simulink model "bola_viga_V_REP_Simulink"  (R2018a)
settings: Solver=ode45  StartTime=0.0  StopTime=144  RelTol=1e-3  EnableMultiTasking=on
undefined symbols (not defined in the file or in its folder): AD, BD, CD, K1, L1, Rep, T, V, V_Rep
libraries: simulink x2, aerolibanimutils x2
settings Model: Creator=HAROLD  LastModifiedBy=HAROLD
settings DataIOCC: LimitDataPoints=on  SaveFormat=Array
settings OptimizationCC: LifeSpan=inf
settings DebuggingCC: SFUnexpectedBacktrackingDiag=warning  SFNoUnconditionalDefaultTransitionDiag=warning  SFExecutionAtInitializationDiag=none
settings HardwareCC: ProdBitPerPointer=32  ProdBitPerSizeT=32  ProdBitPerPtrDiffT=32  ProdLargestAtomicFloat=None  ProdIntDivRoundTo=Undefined  ProdEndianess=Unspecified  ProdWordSize=32  ProdHWDeviceType=32-bit Generic
settings ModelReferenceCC: PropagateSignalLabelsOutOfModel=off
settings CodeAppCC: StateflowObjectComments=on
settings GRTTargetCC: TargetLangStandard=C89/C90 (ANSI)  GeneratePreprocessorConditionals=Disable all
settings ConfigComp: CovMetricSettings=dw  CovHtmlReporting=on  CovSaveCumulativeToWorkspaceVar=on  CovSaveSingleToWorkspaceVar=on  CovExternalEMLEnable=off

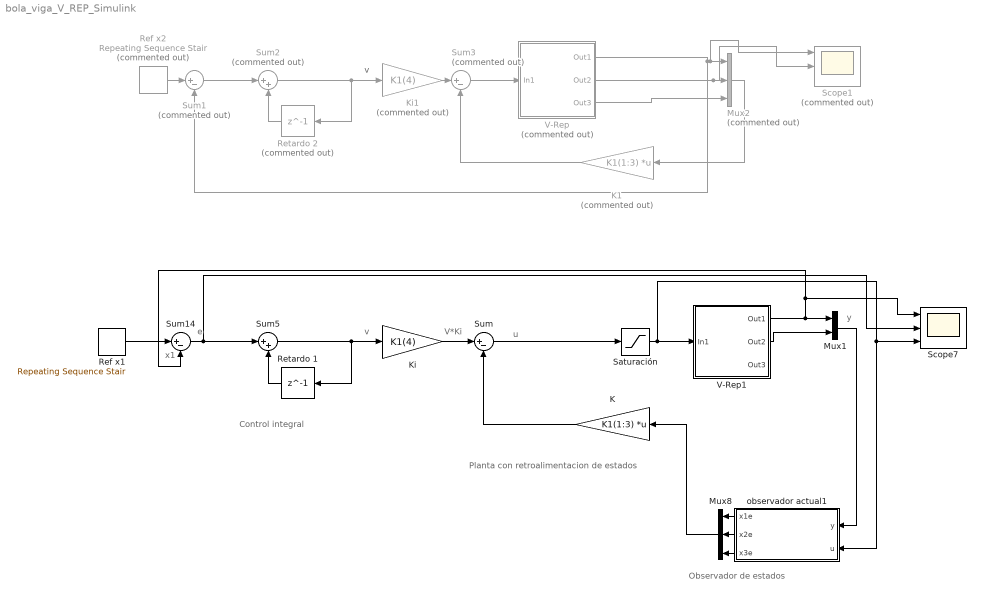
== system bola_viga_V_REP_Simulink ==
  note: v
  note: x1
  note: V*Ki
  note: y
  note: u
  note: v
  note: e
  note: Planta con retroalimentacion de estados
  note: Control integral
  note: Observador de estados
  K : Gain  Gain=K1(1:3)  Multiplication=Matrix(K*u)
  K1 : Gain  Commented=on  Gain=K1(1:3)  Multiplication=Matrix(K*u)
  Ki : Gain  Gain=K1(4)
  Ki1 : Gain  Commented=on  Gain=K1(4)
  Mux1 : Mux  Inputs=2
  Mux2 : Mux  Commented=on  Inputs=3
  Mux8 : Mux  Inputs=3
  Ref x1 : simulink/Sources/Repeating Sequence Stair  OutValues="[0  0.4 -0.4 -0.1 -0.3].'"  tsamp=36*0.8  OutMin=[]  OutMax=[]  OutDataTypeStr=double  OutputDataTypeScalingMode=double  OutDataType=fixdt(0,8)  ConRadixGroup=Best Precision: Vector-wise  OutScaling=2^-12
  Ref x2 : simulink/Sources/Repeating Sequence Stair  Commented=on  OutValues="[0.2  0.4 -0.4 -0.1 -0.3].'"  tsamp=36  OutMin=[]  OutMax=[]  OutDataTypeStr=double  OutputDataTypeScalingMode=double  OutDataType=fixdt(0,8)  ConRadixGroup=Best Precision: Vector-wise  OutScaling=2^-12
  Retardo 1 : Delay  DelayLength=1  SampleTime=T
  Retardo 2 : Delay  Commented=on  DelayLength=1  SampleTime=T
  Saturación : Saturate  UpperLimit=2.11  LowerLimit=-2.11
  Scope1 : Scope  Commented=on  NumInputPorts=3
  Scope7 : Scope  NumInputPorts=3
  Sum : Sum  Inputs=|+-
  Sum1 : Sum  Commented=on  Inputs=|+-
  Sum14 : Sum  Inputs=|+-
  Sum2 : Sum  Commented=on  Inputs=|++
  Sum3 : Sum  Commented=on  Inputs=|+-
  Sum5 : Sum  Inputs=|++
  V-Rep : Subsystem  Commented=on  AncestorBlock=V_Rep/V-Rep  mask(Bloque de V_Rep){Directory=Por Defecto, Parameter1=Bola Viga, Parameter2=T, Parameter3=2, Parameter6=off, Parameter7=3, Parameter8=C:\Program Files\V-REP3\V-REP_PRO_EDU}
      mask prompts: Directory "Directorio de V-Rep"; Parameter1 "Planta a emular"; Parameter2 "Tiempo de muestreo"; Parameter3 "sfdhg"; Parameter6 "Mostrar error de paso"; Parameter7 "Numero de salidas"; Parameter8 "dasads"
      mask help: Este bloque realiza una conexión con V_Rep, teniendo unas plantas ya preprogramadas para su mayor facilidad.
      mask init:
      | switch get_param(gcb,'Parameter1');
      |     case 'Péndulo de Furuta'
      |         t='3';
      |     case 'Bola Plato'
      |         t='1';
      |     case 'Bola Viga'
      |         t='2';
      |     case 'Otros'
      |         t='0';
      | end
      | set_param(gcb,'Parameter3',t);
      mask TypeOptions Directory: Por Defecto | C:\Program Files\V-REP3\V-REP_PRO_EDU
      mask Callback Directory:
      | DIR=get_param(gcb,'Directory');
      | 
      | if(strcmpi(DIR,'Por Defecto'));
      |     if ismac
      |         DIR='/Applications/V-REP_PRO_EDU_V3_6_2_Mac';
      |     elseif ispc
      |         DIR='C:\Program Files\V-REP3\V-REP_PRO_EDU'
      |     end
      | 
      | end
      | 
      | if ~strcmp(DIR,get_param(gcb,'Parameter8'))
      |     if ~exist(DIR, 'dir')
      |         baseException = MException('MYFUN:BadIndex','MYFUN:BadIndex');
      |         throw(baseException);
      |     else
      | 
      |         if~exist(strcat(DIR,'/credits.txt'), 'file')
      |            baseException = MException('MYFUN:BadIndex','V-Rep no está instalado en el directorio indicado');
      |            throw(baseException);
      |         else
      | 
      |             assignin('base','Path', {['-I' DIR '/programming/common/'],['-I' DIR '/programming/remoteApi/'],['-I' DIR '/programming/include/']});
      |             save('Path.mat','Path'),
      |             load('Path.mat');
      |             mex('-v',Path{1,1},Path{1,2},Path{1,3},'v.c','v_Rep_wrapper.c');
      |         end
      |     end
      |     set_param(gcb,'Parameter8',DIR)
      | end
      mask TypeOptions Parameter1: Péndulo de Furuta | Bola Plato | Bola Viga | Otros
      mask Callback Parameter1:
      | NM=str2num(get_param([gcb '/Demux2'],'Outputs'));
      | i = Simulink.Mask.get(gcb);
      | i=i.Parameters(6);
      | switch get_param(gcb,'Parameter1')
      |     case 'Péndulo de Furuta'
      |         i.set('Enabled','off');
      |         N=4;
      |     case 'Bola Plato'
      |         i.set('Enabled','off');
      |         N=3;
      |     case 'Bola Viga'
      |         i.set('Enabled','off');
      |         N=3;
      |     case 'Otros'
      |         i.set('Enabled','on');
      |         N=NM;
      | end
      | set_param(gcb,'Parameter7',num2str(N));
      | if N~=NM
      |     if getSimulinkBlockHandle([gcb '/Out' num2str(NM+1,'%01d')])~=-1 & strcmp(get_param(gcb,'Parameter6'),'on')
      |          delete_line(gcb,'Simulation Pace/1',['Out' num2str(NM+1,'%01d') '/1']);
      |          delete_block([gcb '/Out' num2str(NM+1,'%01d')]);
      |     end
      |     if N<NM
      |         for i=NM:-1:N+1
      |             delete_line(gcb,['Demux2/' num2str(i,'%01d')],['Out' num2str(i,'%01d') '/1']);
      |             delete_block([gcb '/Out' num2str(i,'%01d')]);
      |         end
      |                 set_param([gcb '/Demux2'],'Outputs',num2str(N))
      |     else
      |         set_param([gcb '/Demux2'],'Outputs',num2str(N))
      |         for i=NM+1:N
      |             add_block('simulink/Commonly Used Blocks/Out1',[gcb '/Out'  num2str(i,'%01d')]);
      |             add_line(gcb,['Demux2/' num2str(i,'%01d')],['Out' num2str(i,'%01d') '/1']);
      |         end
      |     end
      | 
      |     if getSimulinkBlockHandle([gcb '/Out' num2str(N+1,'%01d')]) ==-1 & strcmp(get_param(gcb,'Parameter6'),'on')
      |          add_block('simulink/Commonly Used Blocks/Out1',[gcb '/Out' num2str(N+1,'%01d')]);
      |          add_line(gcb,'Simulation Pace/1',['Out' num2str(N+1,'%01d') '/1']);
      |     end
      | 
      | end
      mask Callback Parameter6:
      | NM=get_param([gcb '/Demux2'],'Outputs');
      | if strcmp(get_param(gcb,'Parameter6'),'on')
      |     set_param([gcb '/Simulation Pace'],'OutputPaceError',get_param(gcb,'Parameter6'));
      |     if getSimulinkBlockHandle([gcb '/Out' NM+1]) ==-1
      |         add_block('simulink/Commonly Used Blocks/Out1',[gcb '/Out' NM+1]);
      |         add_line(gcb,'Simulation Pace/1',['Out' NM+1 '/1']);
      |     end
      | else
      |     if getSimulinkBlockHandle([gcb '/Out' NM+1])  ~=-1
      |         delete_line(gcb,'Simulation Pace/1',['Out' NM+1 '/1']);
      |         delete_block([gcb '/Out' NM+1]);
      |     end
      |     set_param([gcb '/Simulation Pace'],'OutputPaceError',get_param(gcb,'Parameter6'));
      | end
      mask Callback Parameter7:
      | NM=str2num(get_param([gcb '/Demux2'],'Outputs'));
      | N=str2num(get_param(gcb,'Parameter7'));
      | if N~=NM
      |     if getSimulinkBlockHandle([gcb '/Out' num2str(NM+1,'%01d')])~=-1 & strcmp(get_param(gcb,'Parameter6'),'on')
      |         delete_line(gcb,'Simulation Pace/1',['Out' num2str(NM+1,'%01d') '/1']);
      |         delete_block([gcb '/Out' num2str(NM+1,'%01d')]);
      |     end
      |     if N<NM
      |         for i=NM:-1:N+1
      |             delete_line(gcb,['Demux2/' num2str(i,'%01d')],['Out' num2str(i,'%01d') '/1']);
      |             delete_block([gcb '/Out' num2str(i,'%01d')]);
      |         end
      |     else
      |         set_param([gcb '/Demux2'],'Outputs',num2str(N))
      |         for i=NM+1:N
      |             add_block('simulink/Commonly Used Blocks/Out1',[gcb '/Out'  num2str(i,'%01d')]);
      |             add_line(gcb,['Demux2/' num2str(i,'%01d')],['Out' num2str(i,'%01d') '/1']);
      |         end
      |     end
      |     if getSimulinkBlockHandle([gcb '/Out' num2str(N+1,'%01d')]) ==-1 & strcmp(get_param(gcb,'Parameter6'),'on')
      |         add_block('simulink/Commonly Used Blocks/Out1',[gcb '/Out' num2str(N+1,'%01d')]);
      |         add_line(gcb,'Simulation Pace/1',['Out' num2str(N+1,'%01d') '/1']);
      |     end
      |     set_param([gcb '/Demux2'],'Outputs',num2str(N))
      | end
      mask DialogControl Container3 Prompt: Directorio V-Rep
      mask DialogControl Control2 Prompt: Buscar
      mask DialogControl Control2 Callback:
      | path = uigetdir();
      | if path~=0
      | 
      |     p=Simulink.Mask.get(gcb)
      |     p.Parameters(1).TypeOptions={'Por Defecto',path};
      |     set_param(gcb,'Directory',1)
      |     if ~exist(path, 'dir')
      |         baseException = MException('V-Rep no está instalado en el directorio indicado','El directorio no existe');
      |         throw(baseException);
      |     else
      | 
      |         if~exist(strcat(path,'/credits.txt'), 'file')
      |            baseException = MException('MYFUN:BadIndex','V-Rep no está instalado en el directorio indicado');
      |            throw(baseException);
      |         else
      |             assignin('base','Path', {['-I' DIR '/programming/common/'],['-I' DIR '/programming/remoteApi/'],['-I' DIR '/programming/include/']});
      |             save('Path.mat','Path')
      |             load('Path.mat');
      |             mex('-v',Path{1,1},Path{1,2},Path{1,3},'v.c','v_Rep_wrapper.c');
      |         end
      |     end
      | end
      mask DialogControl ParameterGroupVar Prompt: Parametros
      mask DialogControl Container5 Prompt: Otros
      mask Display:
      | disp('V-Rep');
      | port_label('input', 1, 'u');
      | N= get_param(gcb,'Parameter7');
      | 
      | for i=1:str2num(N)
      |     port_label('output',i,['x' num2str(i)]);
      | end
      | if strcmp(get_param(gcb,'Parameter6'),'on')
      |     port_label('output',str2num(N)+1, 'Error');
      | end
  V-Rep1 : Subsystem  AncestorBlock=V_Rep/V-Rep  mask(Bloque de V_Rep){Directory=Por Defecto, Parameter1=Bola Viga, Parameter2=T, Parameter3=2, Parameter6=off, Parameter7=3, Parameter8=C:\Program Files\V-REP3\V-REP_PRO_EDU}
      mask prompts: Directory "Directorio de V-Rep"; Parameter1 "Planta a emular"; Parameter2 "Tiempo de muestreo"; Parameter3 "sfdhg"; Parameter6 "Mostrar error de paso"; Parameter7 "Numero de salidas"; Parameter8 "dasads"
      mask help: Este bloque realiza una conexión con V_Rep, teniendo unas plantas ya preprogramadas para su mayor facilidad.
      mask init: same as bola_viga_V_REP_Simulink/V-Rep
      mask TypeOptions Directory: Por Defecto | C:\Program Files\V-REP3\V-REP_PRO_EDU
      mask Callback Directory:
      | DIR=get_param(gcb,'Directory');
      | 
      | if(strcmpi(DIR,'Por Defecto'));
      |     if ismac
      |         DIR='/Applications/V-REP_PRO_EDU_V3_6_2_Mac';
      |     elseif ispc
      |         DIR='C:\Program Files\V-REP3\V-REP_PRO_EDU'
      |     end
      | 
      | end
      | 
      | if ~strcmp(DIR,get_param(gcb,'Parameter8'))
      |     if ~exist(DIR, 'dir')
      |         baseException = MException('MYFUN:BadIndex','MYFUN:BadIndex');
      |         throw(baseException);
      |     else
      | 
      |         if~exist(strcat(DIR,'/credits.txt'), 'file')
      |            baseException = MException('MYFUN:BadIndex','V-Rep no está instalado en el directorio indicado');
      |            throw(baseException);
      |         else
      | 
      |             assignin('base','Path', {['-I' DIR '/programming/common/'],['-I' DIR '/programming/remoteApi/'],['-I' DIR '/programming/include/']});
      |             save('Path.mat','Path'),
      |             load('Path.mat');
      |             mex('-v',Path{1,1},Path{1,2},Path{1,3},'v.c','v_Rep_wrapper.c');
      |         end
      |     end
      |     set_param(gcb,'Parameter8',DIR)
      | end
      mask TypeOptions Parameter1: Péndulo de Furuta | Bola Plato | Bola Viga | Otros
      mask Callback Parameter1:
      | NM=str2num(get_param([gcb '/Demux2'],'Outputs'));
      | i = Simulink.Mask.get(gcb);
      | i=i.Parameters(6);
      | switch get_param(gcb,'Parameter1')
      |     case 'Péndulo de Furuta'
      |         i.set('Enabled','off');
      |         N=4;
      |     case 'Bola Plato'
      |         i.set('Enabled','off');
      |         N=4;
      |     case 'Bola Viga'
      |         i.set('Enabled','off');
      |         N=3;
      |     case 'Otros'
      |         i.set('Enabled','on');
      |         N=NM;
      | end
      | set_param(gcb,'Parameter7',num2str(N));
      | if N~=NM
      |     if getSimulinkBlockHandle([gcb '/Out' num2str(NM+1,'%01d')])~=-1 & strcmp(get_param(gcb,'Parameter6'),'on')
      |          delete_line(gcb,'Simulation Pace/1',['Out' num2str(NM+1,'%01d') '/1']);
      |          delete_block([gcb '/Out' num2str(NM+1,'%01d')]);
      |     end
      |     if N<NM
      |         for i=NM:-1:N+1
      |             delete_line(gcb,['Demux2/' num2str(i,'%01d')],['Out' num2str(i,'%01d') '/1']);
      |             delete_block([gcb '/Out' num2str(i,'%01d')]);
      |         end
      |                 set_param([gcb '/Demux2'],'Outputs',num2str(N))
      |     else
      |         set_param([gcb '/Demux2'],'Outputs',num2str(N))
      |         for i=NM+1:N
      |             add_block('simulink/Commonly Used Blocks/Out1',[gcb '/Out'  num2str(i,'%01d')]);
      |             add_line(gcb,['Demux2/' num2str(i,'%01d')],['Out' num2str(i,'%01d') '/1']);
      |         end
      |     end
      | 
      |     if getSimulinkBlockHandle([gcb '/Out' num2str(N+1,'%01d')]) ==-1 & strcmp(get_param(gcb,'Parameter6'),'on')
      |          add_block('simulink/Commonly Used Blocks/Out1',[gcb '/Out' num2str(N+1,'%01d')]);
      |          add_line(gcb,'Simulation Pace/1',['Out' num2str(N+1,'%01d') '/1']);
      |     end
      | 
      | end
      mask Callback Parameter6:
      | NM=get_param([gcb '/Demux2'],'Outputs');
      | if strcmp(get_param(gcb,'Parameter6'),'on')
      |     set_param([gcb '/Simulation Pace'],'OutputPaceError',get_param(gcb,'Parameter6'));
      |     if getSimulinkBlockHandle([gcb '/Out' NM+1]) ==-1
      |         add_block('simulink/Commonly Used Blocks/Out1',[gcb '/Out' NM+1]);
      |         add_line(gcb,'Simulation Pace/1',['Out' NM+1 '/1']);
      |     end
      | else
      |     if getSimulinkBlockHandle([gcb '/Out' NM+1])  ~=-1
      |         delete_line(gcb,'Simulation Pace/1',['Out' NM+1 '/1']);
      |         delete_block([gcb '/Out' NM+1]);
      |     end
      |     set_param([gcb '/Simulation Pace'],'OutputPaceError',get_param(gcb,'Parameter6'));
      | end
      mask Callback Parameter7:
      | NM=str2num(get_param([gcb '/Demux2'],'Outputs'));
      | N=str2num(get_param(gcb,'Parameter7'));
      | if N~=NM
      |     if getSimulinkBlockHandle([gcb '/Out' num2str(NM+1,'%01d')])~=-1 & strcmp(get_param(gcb,'Parameter6'),'on')
      |         delete_line(gcb,'Simulation Pace/1',['Out' num2str(NM+1,'%01d') '/1']);
      |         delete_block([gcb '/Out' num2str(NM+1,'%01d')]);
      |     end
      |     if N<NM
      |         for i=NM:-1:N+1
      |             delete_line(gcb,['Demux2/' num2str(i,'%01d')],['Out' num2str(i,'%01d') '/1']);
      |             delete_block([gcb '/Out' num2str(i,'%01d')]);
      |         end
      |     else
      |         set_param([gcb '/Demux2'],'Outputs',num2str(N))
      |         for i=NM+1:N
      |             add_block('simulink/Commonly Used Blocks/Out1',[gcb '/Out'  num2str(i,'%01d')]);
      |             add_line(gcb,['Demux2/' num2str(i,'%01d')],['Out' num2str(i,'%01d') '/1']);
      |         end
      |     end
      |     if getSimulinkBlockHandle([gcb '/Out' num2str(N+1,'%01d')]) ==-1 & strcmp(get_param(gcb,'Parameter6'),'on')
      |         add_block('simulink/Commonly Used Blocks/Out1',[gcb '/Out' num2str(N+1,'%01d')]);
      |         add_line(gcb,'Simulation Pace/1',['Out' num2str(N+1,'%01d') '/1']);
      |     end
      |     set_param([gcb '/Demux2'],'Outputs',num2str(N))
      | end
      mask DialogControl Container3 Prompt: Directorio V-Rep
      mask DialogControl Control2 Prompt: Buscar
      mask DialogControl Control2 Callback:
      | path = uigetdir();
      | if path~=0
      | 
      |     p=Simulink.Mask.get(gcb)
      |     p.Parameters(1).TypeOptions={'Por Defecto',path};
      |     set_param(gcb,'Directory',1)
      |     if ~exist(path, 'dir')
      |         baseException = MException('V-Rep no está instalado en el directorio indicado','El directorio no existe');
      |         throw(baseException);
      |     else
      | 
      |         if~exist(strcat(path,'/credits.txt'), 'file')
      |            baseException = MException('MYFUN:BadIndex','V-Rep no está instalado en el directorio indicado');
      |            throw(baseException);
      |         else
      |             assignin('base','Path', {['-I' DIR '/programming/common/'],['-I' DIR '/programming/remoteApi/'],['-I' DIR '/programming/include/']});
      |             save('Path.mat','Path')
      |             load('Path.mat');
      |             mex('-v',Path{1,1},Path{1,2},Path{1,3},'v.c','v_Rep_wrapper.c');
      |         end
      |     end
      | end
      mask DialogControl ParameterGroupVar Prompt: Parametros
      mask DialogControl Container5 Prompt: Otros
      mask Display:
      | disp('V-Rep');
      | port_label('input', 1, 'u');
      | N= get_param(gcb,'Parameter7');
      | 
      | for i=1:str2num(N)
      |     port_label('output',i,['x' num2str(i)]);
      | end
      | if strcmp(get_param(gcb,'Parameter6'),'on')
      |     port_label('output',str2num(N)+1, 'Error');
      | end
  observador actual1 : Subsystem
  wires:
  Ref x2/1 -> Sum1/1
  Retardo 2/1 -> Sum2/2
  Sum2/1 -> Retardo 2/1, Ki1/1
  Sum1/1 -> Sum2/1
  Ki1/1 -> Sum3/1
  K1/1 -> Sum3/2
  Sum3/1 -> V-Rep/1(In1)
  V-Rep/1(Out1) -> Sum1/2, Scope1/1, Mux2/1
  V-Rep/2(Out2) -> Scope1/2, Mux2/2
  V-Rep/3(Out3) -> Mux2/3
  Mux2/1 -> K1/1
  Sum/1 -> Saturación/1
  Retardo 1/1 -> Sum5/2
  Sum5/1 -> Retardo 1/1, Ki/1
  Ki/1 -> Sum/1
  Sum14/1 -> Sum5/1, Scope7/2
  Ref x1/1 -> Sum14/1
  K/1 -> Sum/2
  V-Rep1/1(Out1) -> Scope7/1, Sum14/2, Mux1/1
  Saturación/1 -> V-Rep1/1(In1), observador actual1/2(u), Scope7/3
  observador actual1/1(x1e) -> Mux8/1
  observador actual1/2(x2e) -> Mux8/2
  Mux8/1 -> K/1
  V-Rep1/2(Out2) -> Mux1/2
  Mux1/1 -> observador actual1/1(y)
  observador actual1/3(x3e) -> Mux8/3

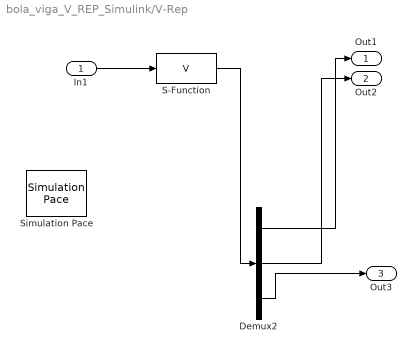
== system bola_viga_V_REP_Simulink/V-Rep ==
  In1 : Inport
  Demux2 : Demux  Outputs=3
  S-Function : S-Function  FunctionName=V  Parameters=Parameter3,Parameter2,Parameter7  SFunctionModules=V_wrapper  SFunctionDeploymentMode=off  EnableBusSupport=off
  Simulation Pace : aerolibanimutils/Simulation Pace  SimulationPace=1  SleepMode=MATLAB Thread  OutputPaceError=off  SampleTime=Parameter2
  Out1 : Outport
  Out2 : Outport  Port=2
  Out3 : Outport  Port=3
  wires:
  Demux2/3 -> Out3/1
  Demux2/2 -> Out2/1
  In1/1 -> S-Function/1
  S-Function/1 -> Demux2/1
  Demux2/1 -> Out1/1

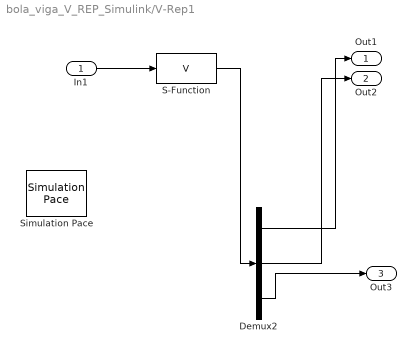
== system bola_viga_V_REP_Simulink/V-Rep1 ==
  In1 : Inport
  Demux2 : Demux  Outputs=3
  S-Function : S-Function  FunctionName=V  Parameters=Parameter3,Parameter2,Parameter7  SFunctionModules=V_wrapper  SFunctionDeploymentMode=off  EnableBusSupport=off
  Simulation Pace : aerolibanimutils/Simulation Pace  SimulationPace=1  SleepMode=MATLAB Thread  OutputPaceError=off  SampleTime=Parameter2
  Out1 : Outport
  Out2 : Outport  Port=2
  Out3 : Outport  Port=3
  wires:
  Demux2/3 -> Out3/1
  Demux2/2 -> Out2/1
  In1/1 -> S-Function/1
  S-Function/1 -> Demux2/1
  Demux2/1 -> Out1/1

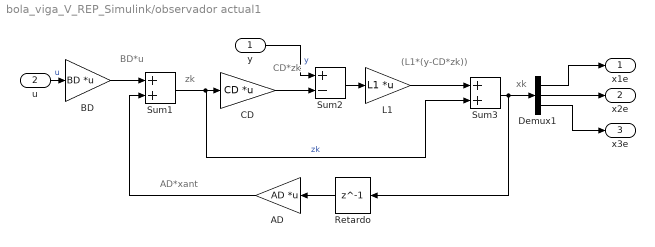
== system bola_viga_V_REP_Simulink/observador actual1 ==
  note: xk
  note: (L1*(y-CD*zk))
  note: CD*zk
  note: AD*xant
  note: BD*u
  note: zk
  y : Inport
  u : Inport  Port=2
  AD : Gain  Gain=AD  Multiplication=Matrix(K*u)
  BD : Gain  Gain=BD  Multiplication=Matrix(K*u)
  CD : Gain  Gain=CD  Multiplication=Matrix(K*u)
  Demux1 : Demux  Outputs=3
  L1 : Gain  Gain=L1  Multiplication=Matrix(K*u)
  Retardo : Delay  DelayLength=1  InitialCondition=[0 0 0]  SampleTime=T
  Sum1 : Sum
  Sum2 : Sum  Inputs=+-
  Sum3 : Sum
  x1e : Outport
  x2e : Outport  Port=2
  x3e : Outport  Port=3
  wires:
  Demux1/1 -> x1e/1
  Demux1/2 -> x2e/1
  Demux1/3 -> x3e/1
  Sum2/1 -> L1/1
  Sum1/1 -> Sum3/2, CD/1  "zk"
  Sum3/1 -> Demux1/1, Retardo/1
  BD/1 -> Sum1/1
  AD/1 -> Sum1/2
  L1/1 -> Sum3/1
  CD/1 -> Sum2/2
  Retardo/1 -> AD/1
  u/1 -> BD/1  "u"
  y/1 -> Sum2/1  "y"
